simulink model "rx_udp"  (R2019a)
settings: Solver=FixedStepAuto  StartTime=0.0  StopTime=Inf  FixedStep=0.001  RelTol=1e-3
PostLoadFcn:
  | if any(exist('dsrtsu_mdlpostloadfcn', 'file') ~= 0), dsrtsu_mdlpostloadfcn('Execute', bdroot); end
libraries: dsaV2xLibraryAux x2, dsaV2xAsn1Library x1, dsaV2xLibrary x1, veos_ethernet_blockset x1
PreSaveFcn:
  | , if any(exist('dsmpb_private', 'file') ~= 0), dsmpb_private('dsmpb_mdlclblib', 'PreSave', bdroot); end,
CloseFcn:
  | , if any(exist('dsmpb_private', 'file') ~= 0), dsmpb_private('dsmpb_mdlclblib', 'Close', bdroot); end,
settings Model: RTICANMMDATA=struct('GeneralSetupData',struct('modelroot','C:\Users\FHAachenHIL\Desktop\Multi_Message_TX','generalsettings',struct('filesettings',struct('destfolder',struct('Name','RTICANMM_FILES','Check',1),'buildfolder',struct('Name','.','Check',1),'AbsDestfolder',struct('Name','C:\Users\FHAachenHIL\Desktop\Multi_Message_TX\RTICANMM_FILES'),'AbsBuildfolder',struct('Name','C:\Users\FHAachenHIL\Desktop\Multi_Message_TX'))),'options',struct('addpaths',1,'rmpaths',1,'addtrcexclusion',logical(1),'cannavigator',struct('checkmonitoring',0),'show_usrtrc',0,'use_usrtrc',0),'advanced',struct('options',ones(1,100)),'MPSetup',{{}},'RTI',struct('Type','DSRT','Ver','4.1','Date','02-May-2019'),'modelname','','block','untitled'))  DSRTSU_INTERNAL_RTIFPGA=130  DSMPB_ID_DATA={'17',struct('BlockId','ce67a496-d825-4533-83aa-cfdb9bca819b','SignalIds',{{'4f09f7b1-0df2-45d5-94ea-0968c0cc2653','75673753-4807-4aba-9152-07f64725ffff','f5b87971-be41-4a77-9852-6fd8f5d2bf57','3fb2f5ec-d680-4aa2-8664-9f8ef777f0de','c28a46f3-5b17-413c-bffd-903dfd89be5b'}})}  Creator=FHAachenHIL  LastModifiedBy=aydin
settings OptimizationCC: BlockReduction=off  ConditionallyExecuteInputs=off  OptimizeBlockIOStorage=off  BufferReuse=off  GlobalBufferReuse=off  ExpressionFolding=off  LocalBlockOutputs=off  OptimizeDataStoreBuffers=off  BusAssignmentInplaceUpdate=off
settings DebuggingCC: InheritedTsInSrcMsg=none  TasksWithSamePriorityMsg=none
settings HardwareCC: ProdBitPerPointer=32  ProdBitPerSizeT=32  ProdBitPerPtrDiffT=32  ProdLargestAtomicInteger=Integer  ProdWordSize=32  ProdHWDeviceType=Custom Processor->Custom
settings SFSimCC: MATLABDynamicMemAlloc=off
settings RTWCC: SystemTargetFile=dsrt.tlc  GenCodeOnly=on  MakeCommand=make_dsrt  TemplateMakefile=dsrt_default_tmf  Description=dSPACE Run-Time Target (for VEOS and ConfigurationDesk)  RTWVerbose=off
settings STFCustomTargetCC: TargetLangStandard=C99 (ISO)  ParMdlRefBuildCompliant=on  GRTInterface=off  SystemTargetFile=dsrt.tlc
settings GRTTargetCC: CompOptLevelCompliant=off  ConcurrentExecutionCompliant=off  CombineOutputUpdateFcns=off  MatFileLogging=off  CPPClassGenCompliant=off  UseToolchainInfoCompliant=off

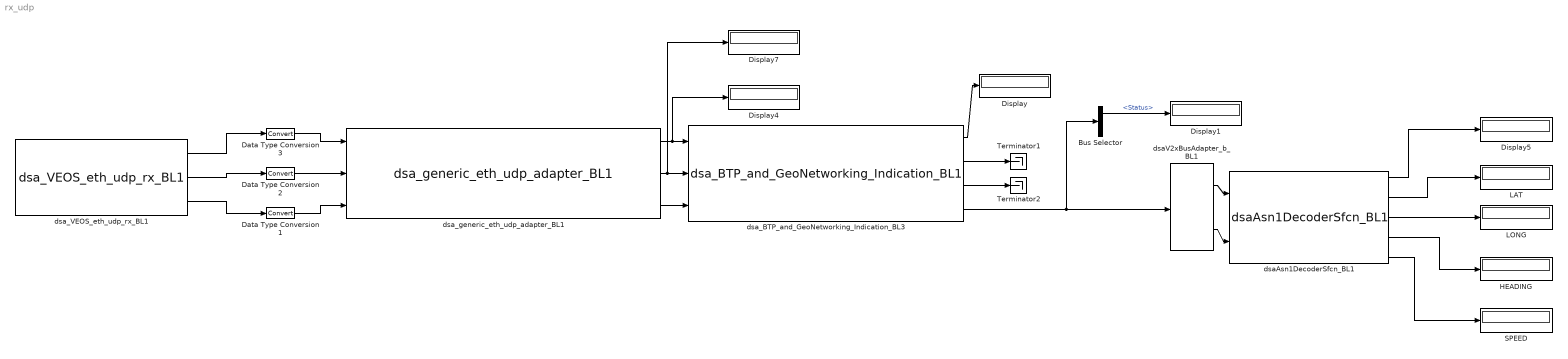
== system rx_udp ==
  Bus Selector : BusSelector  OutputSignals=Status,Length
  Data Type Conversion1 : DataTypeConversion
  Data Type Conversion2 : DataTypeConversion
  Data Type Conversion3 : DataTypeConversion
  Display{,1,4..5,7} (5 alike) : Display
  HEADING : Display
  LAT : Display
  LONG : Display
  SPEED : Display
  Terminator1 : Terminator
  Terminator2 : Terminator
  dsaAsn1DecoderSfcn_BL1 : dsaV2xAsn1Library/dsaAsn1DecoderSfcn_BL1  xml="<?xml version=\"1.0\" encoding=\"utf-8\"?><ArrayOfEntry xmlns:xsd=\"http://www.w3.org/2001/XMLSchema\" xmlns:xsi=\"http://www.w3.org/2001/XMLSchema-instance\"><Entry><Name>latitude</Name><Xpath>/CAM/cam/camParameters/basicContainer/referencePosition/latitude</Xpath><OutputBehaviour>Number</OutputBehaviour><MaxLength>512</MaxLength><Invalid>-1</Invalid></Entry><Entry><Name>longitude</Name><Xpath>/CAM/cam/camParameters/basicContainer/referencePosition/longitude</Xpath><OutputBehaviour>Number</OutputBehaviour><MaxLength>512</MaxLength><Invalid>-1</Invalid></Entry><Entry><Name>heading</Name><Xpath>/CAM/cam/camParameters/highFrequencyContainer/basicVehicleContainerHighFrequency/heading</Xpath><OutputBehaviour>Number</OutputBehaviour><MaxLength>512</MaxLength><Invalid>-1</Invalid></Entry><Entry><Name>speed</Name><Xpath>/CAM/cam/camParameters/highFrequencyContainer/basicVehicleContainerHighFrequency/speed</Xpath><OutputBehaviour>Number</OutputBehaviour><MaxLength>512</MaxLength><Invalid>-1</Invalid></Entry></ArrayOfEntry>"  typeStr=CAM (ETSI EN 302 637-2 v1.3.2)  encDecType=1  sampleTime=-1
      settings: AttributesFormatString=%<typeStr>  SourceProductName=dSPACE [SOL] V2X ASN.1 Blockset
  dsaV2xBusAdapter_b_BL1 : dsaV2xLibraryAux/dsaV2xBusAdapter_b_BL1  SystemSampleTime=-1
  dsa_BTP_and_GeoNetworking_Indication_BL3 : dsaV2xLibrary/dsa_BTP_and_GeoNetworking_Indication_BL1  btpType=BTP-B (non-interactive)  destinationPort=CAM  sourcePort=CAM  destinationPortInfo=0 (default)  packetTransportType=Topologically Scoped Brodcast  securityProfile=UNSECURED  scf=on  scfMode=don't care  channelOffload=on  channelOffloadMode=don't care  tcId=High-priority DENM  tcIdMode=don't care  style=CohdaWireless MK5
      settings: SourceProductName=dSPACE [SOL] V2X Blockset
  dsa_VEOS_eth_udp_rx_BL1 : veos_ethernet_blockset/dsa_VEOS_eth_udp_rx_BL1  paramRxPort=37008  paramRxBlockingTime=1  cBoxRemoteIp=off  rx_ip_1=192  rx_ip_2=168  rx_ip_3=1  rx_ip_4=10  paramMaximumRxMessageSize=1472
      settings: SourceProductName=dSPACE [SOL] VEOS Ethernet Blockset
  dsa_generic_eth_udp_adapter_BL1 : dsaV2xLibraryAux/dsa_generic_eth_udp_adapter_BL1  style=SCALEXIO Ethernet Solution  direction=Rx  maxSize=1472
  wires:
  dsa_generic_eth_udp_adapter_BL1/3 -> dsa_BTP_and_GeoNetworking_Indication_BL3/3
  Data Type Conversion3/1 -> dsa_generic_eth_udp_adapter_BL1/1
  dsa_VEOS_eth_udp_rx_BL1/1 -> Data Type Conversion3/1
  dsaAsn1DecoderSfcn_BL1/5 -> SPEED/1
  dsaAsn1DecoderSfcn_BL1/4 -> HEADING/1
  dsaV2xBusAdapter_b_BL1/2 -> dsaAsn1DecoderSfcn_BL1/2
  dsaAsn1DecoderSfcn_BL1/3 -> LONG/1
  dsaAsn1DecoderSfcn_BL1/2 -> LAT/1
  dsa_VEOS_eth_udp_rx_BL1/3 -> Data Type Conversion1/1
  dsaAsn1DecoderSfcn_BL1/1 -> Display5/1
  dsa_generic_eth_udp_adapter_BL1/1 -> Display4/1, dsa_BTP_and_GeoNetworking_Indication_BL3/1
  dsaV2xBusAdapter_b_BL1/1 -> dsaAsn1DecoderSfcn_BL1/1
  dsa_generic_eth_udp_adapter_BL1/2 -> Display7/1, dsa_BTP_and_GeoNetworking_Indication_BL3/2
  Data Type Conversion1/1 -> dsa_generic_eth_udp_adapter_BL1/3
  Data Type Conversion2/1 -> dsa_generic_eth_udp_adapter_BL1/2
  dsa_VEOS_eth_udp_rx_BL1/2 -> Data Type Conversion2/1
  dsa_BTP_and_GeoNetworking_Indication_BL3/1 -> Display/1
  dsa_BTP_and_GeoNetworking_Indication_BL3/2 -> Terminator1/1
  dsa_BTP_and_GeoNetworking_Indication_BL3/3 -> Terminator2/1
  Bus Selector/1 -> Display1/1  "<Status>"
  dsa_BTP_and_GeoNetworking_Indication_BL3/4 -> Bus Selector/1, dsaV2xBusAdapter_b_BL1/1
